simulink model "clockwise_sim"  (R2021a)
settings: Solver=VariableStepAuto  StartTime=0.0  StopTime=20  RelTol=1e-3
undefined symbols (not defined in the file): g, I, l, m
libraries: simulink x1
settings Model: Creator=1  LastModifiedBy=1

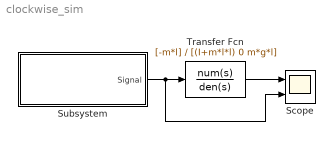
== system clockwise_sim ==
  Scope : Scope  NumInputPorts=2
  Subsystem : Subsystem  mask{st=0.005, amp=1, freq=1}
      mask prompts: st "Sample time(s)"; amp "Amplitude"; freq "Frequency(Hz)"
      mask help: Sample time：必须和系统周期保持一致
      mask Display: disp('自定义方波信号')
  Transfer Fcn : TransferFcn  Numerator=[-m*l]  Denominator=[(I+m*l*l) 0 m*g*l]
  wires:
  Transfer Fcn/1 -> Scope/1
  Subsystem/1(Signal) -> Transfer Fcn/1, Scope/2

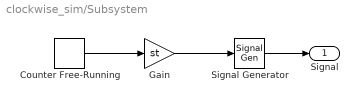
== system clockwise_sim/Subsystem ==
  Counter Free-Running : simulink/Sources/Counter Free-Running  NumBits=32  tsamp=-1
  Gain : Gain  Gain=st  OutDataTypeStr=double
  Signal Generator : SignalGenerator  WaveForm=square  TimeSource=Use external signal  Amplitude=amp  Frequency=freq
  Signal : Outport
  wires:
  Counter Free-Running/1 -> Gain/1
  Signal Generator/1 -> Signal/1
  Gain/1 -> Signal Generator/1
